simulink model "test_urarm_movetool"
settings: Solver=ode45  StartTime=0.0  StopTime=10.0  RelTol=1e-3
libraries: urarm_simulink x1
settings Model: Creator=fkzhang  LastModifiedBy=Sunniva
settings DataIOCC: LimitDataPoints=on  SaveFormat=Array  SignalLoggingSaveFormat=ModelDataLogs  ReturnWorkspaceOutputs=off
settings OptimizationCC: LifeSpan=inf  SimCompilerOptimization=Off
settings DebuggingCC: UnderspecifiedInitializationDetection=Classic  MergeDetectMultiDrivingBlocksExec=none  SolverPrmCheckMsg=warning  MultiTaskDSMMsg=warning  MultiTaskCondExecSysMsg=none  FcnCallInpInsideContextMsg=Enable All  FrameProcessingCompatibilityMsg=warning  StrictBusMsg=None  SFUnexpectedBacktrackingDiag=warning  SFNoUnconditionalDefaultTransitionDiag=warning
settings HardwareCC: ProdBitPerPointer=32  ProdLargestAtomicFloat=None  ProdIntDivRoundTo=Undefined  ProdEndianess=Unspecified  ProdWordSize=32  ProdHWDeviceType=32-bit Generic
settings ModelReferenceCC: PropagateSignalLabelsOutOfModel=off
settings SFSimCC: SimUseLocalCustomCode=off
settings RTWCC: RTWUseLocalCustomCode=off  IncludeERTFirstTime=on  RTWCompilerOptimization=Off
settings GRTTargetCC: CodeReplacementLibrary=ANSI_C  GeneratePreprocessorConditionals=Disable all  CPPClassGenCompliant=off

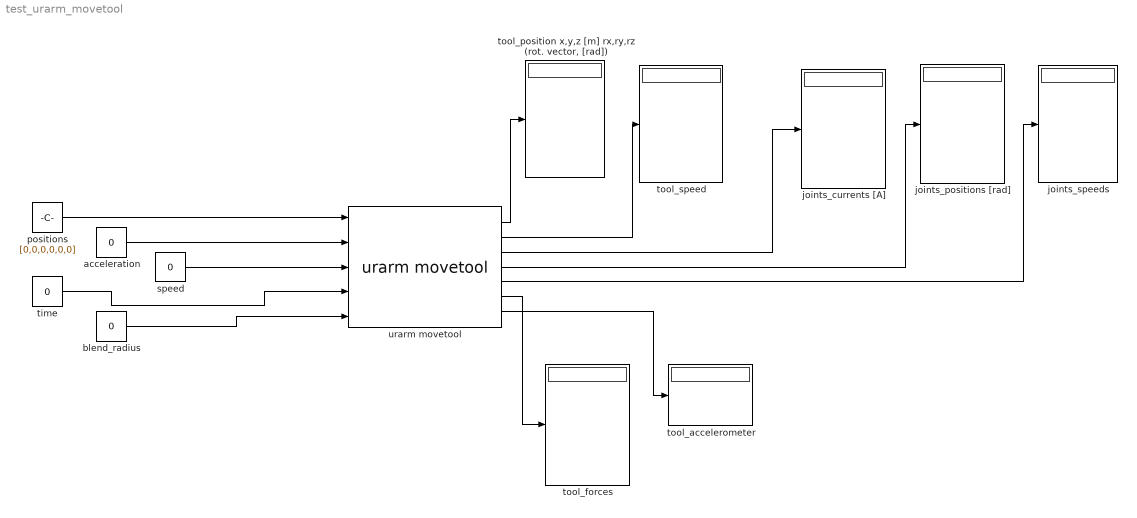
== system test_urarm_movetool ==
  acceleration : Constant  Value=0
  blend_radius : Constant  Value=0
  joints_currents [A] : Display
  joints_positions [rad] : Display
  joints_speeds : Display
  positions : Constant  Value=[0,0,0,0,0,0]
  speed : Constant  Value=0
  time : Constant  Value=0
  tool_accelerometer : Display
  tool_forces : Display
  "tool_position x,y,z [m] rx,ry,rz (rot. vector, [rad])" : Display
  tool_speed : Display
  urarm movetool : urarm_simulink/urarm movetool  Ts=1/100
  wires:
  urarm movetool/3 -> joints_currents [A]/1
  urarm movetool/1 -> "tool_position x,y,z [m] rx,ry,rz (rot. vector, [rad])"/1
  urarm movetool/2 -> tool_speed/1
  urarm movetool/4 -> joints_positions [rad]/1
  urarm movetool/5 -> joints_speeds/1
  urarm movetool/6 -> tool_forces/1
  urarm movetool/7 -> tool_accelerometer/1
  speed/1 -> urarm movetool/3
  acceleration/1 -> urarm movetool/2
  positions/1 -> urarm movetool/1
  time/1 -> urarm movetool/4
  blend_radius/1 -> urarm movetool/5
